simulink model "pmsm"  (R2014b)
settings: Solver=ode45  StartTime=0.0  StopTime=10.0  RelTol=1e-3
undefined symbols (not defined in the file): flux, J, Ld, Lq, Pn, R
settings Model: CovSFcnEnable=on  Creator=Lei  LastModifiedBy=Lei
settings DataIOCC: SignalLoggingSaveFormat=ModelDataLogs  SignalLoggingName=sigsOut
settings DebuggingCC: SaveWithParameterizedLinksMsg=none  UnderspecifiedInitializationDetection=Classic  MergeDetectMultiDrivingBlocksExec=none  SignalResolutionControl=TryResolveAllWithWarning  SolverPrmCheckMsg=none  MultiTaskDSMMsg=warning  MultiTaskCondExecSysMsg=none  FrameProcessingCompatibilityMsg=error  StrictBusMsg=None
settings HardwareCC: TargetUnknown=on
settings GRTTargetCC: CombineOutputUpdateFcns=off  GRTInterface=on

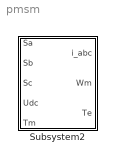
== system pmsm ==
  Subsystem2 : Subsystem

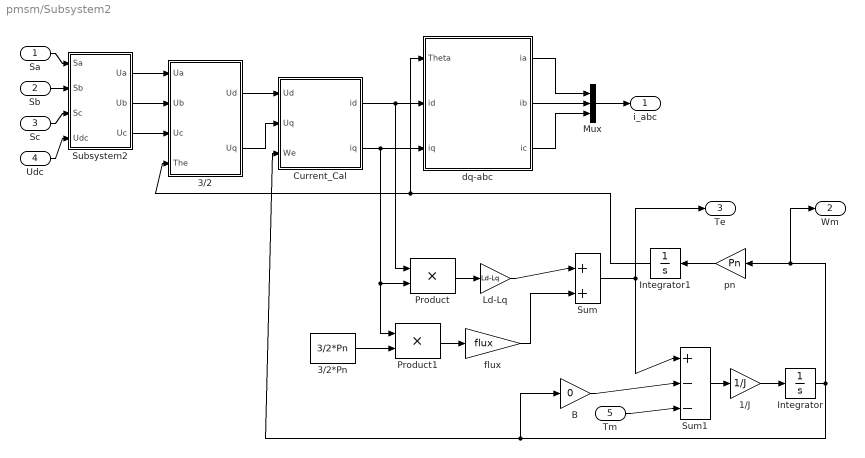
== system pmsm/Subsystem2 ==
  Sa : Inport
  Sb : Inport  Port=2
  Sc : Inport  Port=3
  Udc : Inport  Port=4
  Tm : Inport  Port=5
  1/J : Gain  Gain=1/J  SaturateOnIntegerOverflow=on  OutDataTypeStr=Inherit: Same as input  ParamDataTypeStr=Inherit: Same as input
  3/2 : Subsystem
  3/2*Pn : Constant  Value=3/2*Pn
  B : Gain  Gain=0  SaturateOnIntegerOverflow=on  OutDataTypeStr=Inherit: Same as input  ParamDataTypeStr=Inherit: Same as input
  Current_Cal : Subsystem
  Integrator : Integrator
  Integrator1 : Integrator
  Ld-Lq : Gain  Gain=Ld-Lq  SaturateOnIntegerOverflow=on  OutDataTypeStr=Inherit: Same as input  ParamDataTypeStr=Inherit: Same as input
  Mux : Mux  Inputs=3
  Product : Product  SaturateOnIntegerOverflow=on  OutDataTypeStr=Inherit: Same as first input
  Product1 : Product  SaturateOnIntegerOverflow=on  OutDataTypeStr=Inherit: Same as first input
  Subsystem2 : Subsystem
  Sum : Sum  Inputs=|++  SaturateOnIntegerOverflow=on
  Sum1 : Sum  Inputs=|+--  SaturateOnIntegerOverflow=on
  dq-abc : Subsystem
  flux : Gain  Gain=flux  SaturateOnIntegerOverflow=on  OutDataTypeStr=Inherit: Same as input  ParamDataTypeStr=Inherit: Same as input
  pn : Gain  Gain=Pn  SaturateOnIntegerOverflow=on  OutDataTypeStr=Inherit: Same as input  ParamDataTypeStr=Inherit: Same as input
  i_abc : Outport
  Wm : Outport  Port=2
  Te : Outport  Port=3
  wires:
  Current_Cal/1(id) -> dq-abc/2(id), Product/1
  Current_Cal/2(iq) -> dq-abc/3(iq), Product/2, Product1/1
  3/2/1(Ud) -> Current_Cal/1(Ud)
  3/2/2(Uq) -> Current_Cal/2(Uq)
  Subsystem2/1(Ua) -> 3/2/1(Ua)
  Subsystem2/2(Ub) -> 3/2/2(Ub)
  Subsystem2/3(Uc) -> 3/2/3(Uc)
  Product/1 -> Ld-Lq/1
  Ld-Lq/1 -> Sum/1
  Product1/1 -> flux/1
  3/2*Pn/1 -> Product1/2
  flux/1 -> Sum/2
  Sum/1 -> Sum1/1, Te/1
  Tm/1 -> Sum1/3
  B/1 -> Sum1/2
  Sum1/1 -> 1/J/1
  1/J/1 -> Integrator/1
  Integrator/1 -> Current_Cal/3(We), B/1, pn/1, Wm/1
  Integrator1/1 -> 3/2/4(The), dq-abc/1(Theta)
  pn/1 -> Integrator1/1
  dq-abc/1(ia) -> Mux/1
  dq-abc/2(ib) -> Mux/2
  dq-abc/3(ic) -> Mux/3
  Mux/1 -> i_abc/1
  Sb/1 -> Subsystem2/2(Sb)
  Sc/1 -> Subsystem2/3(Sc)
  Udc/1 -> Subsystem2/4(Udc)
  Sa/1 -> Subsystem2/1(Sa)

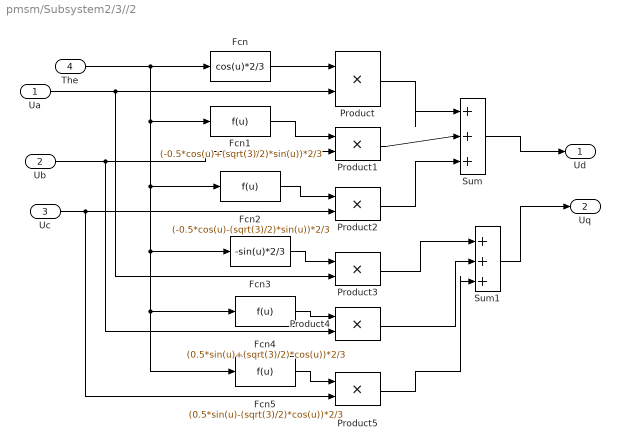
== system pmsm/Subsystem2/3//2 ==
  Ua : Inport
  Ub : Inport  Port=2
  Uc : Inport  Port=3
  The : Inport  Port=4
  Fcn : Fcn  Expr=cos(u)*2/3
  Fcn1 : Fcn  Expr=(-0.5*cos(u)+(sqrt(3)/2)*sin(u))*2/3
  Fcn2 : Fcn  Expr=(-0.5*cos(u)-(sqrt(3)/2)*sin(u))*2/3
  Fcn3 : Fcn  Expr=-sin(u)*2/3
  Fcn4 : Fcn  Expr=(0.5*sin(u)+(sqrt(3)/2)*cos(u))*2/3
  Fcn5 : Fcn  Expr=(0.5*sin(u)-(sqrt(3)/2)*cos(u))*2/3
  Product{,1..5} (6 alike) : Product  SaturateOnIntegerOverflow=on  OutDataTypeStr=Inherit: Same as first input
  Sum : Sum  Inputs=|+++  SaturateOnIntegerOverflow=on
  Sum1 : Sum  Inputs=|+++  SaturateOnIntegerOverflow=on
  Ud : Outport
  Uq : Outport  Port=2
  wires:
  Product/1 -> Sum/1
  Product1/1 -> Sum/2
  Product4/1 -> Sum1/2
  Product5/1 -> Sum1/3
  Sum/1 -> Ud/1
  Fcn/1 -> Product/1
  The/1 -> Fcn1/1, Fcn2/1, Fcn3/1, Fcn5/1, Fcn4/1, Fcn/1
  Ua/1 -> Product/2, Product3/2
  Fcn1/1 -> Product1/1
  Ub/1 -> Product1/2, Product4/2
  Product2/1 -> Sum/3
  Uc/1 -> Product2/2, Product5/2
  Fcn2/1 -> Product2/1
  Sum1/1 -> Uq/1
  Product3/1 -> Sum1/1
  Fcn3/1 -> Product3/1
  Fcn4/1 -> Product4/1
  Fcn5/1 -> Product5/1

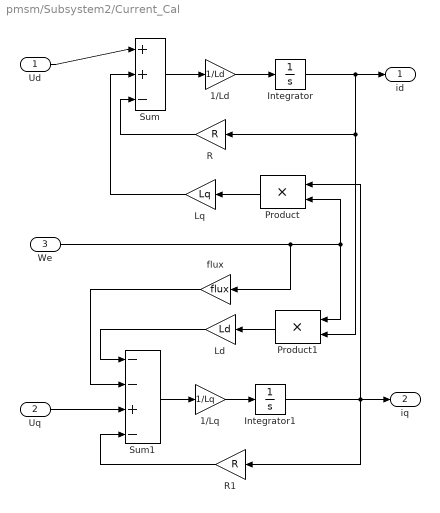
== system pmsm/Subsystem2/Current_Cal ==
  Ud : Inport
  Uq : Inport  Port=2
  We : Inport  Port=3
  1/Ld : Gain  Gain=1/Ld  SaturateOnIntegerOverflow=on  OutDataTypeStr=Inherit: Same as input  ParamDataTypeStr=Inherit: Same as input
  1/Lq : Gain  Gain=1/Lq  SaturateOnIntegerOverflow=on  OutDataTypeStr=Inherit: Same as input  ParamDataTypeStr=Inherit: Same as input
  Integrator : Integrator  InitialCondition=0.01
  Integrator1 : Integrator
  Ld : Gain  Gain=Ld  SaturateOnIntegerOverflow=on  OutDataTypeStr=Inherit: Same as input  ParamDataTypeStr=Inherit: Same as input
  Lq : Gain  Gain=Lq  SaturateOnIntegerOverflow=on  OutDataTypeStr=Inherit: Same as input  ParamDataTypeStr=Inherit: Same as input
  Product : Product  SaturateOnIntegerOverflow=on  OutDataTypeStr=Inherit: Same as first input
  Product1 : Product  SaturateOnIntegerOverflow=on  OutDataTypeStr=Inherit: Same as first input
  R : Gain  Gain=R  SaturateOnIntegerOverflow=on  OutDataTypeStr=Inherit: Same as input  ParamDataTypeStr=Inherit: Same as input
  R1 : Gain  Gain=R  SaturateOnIntegerOverflow=on  OutDataTypeStr=Inherit: Same as input  ParamDataTypeStr=Inherit: Same as input
  Sum : Sum  Inputs=|++-  SaturateOnIntegerOverflow=on
  Sum1 : Sum  Inputs=--+-  SaturateOnIntegerOverflow=on
  flux : Gain  Gain=flux  SaturateOnIntegerOverflow=on  OutDataTypeStr=Inherit: Same as input  ParamDataTypeStr=Inherit: Same as input
  id : Outport
  iq : Outport  Port=2
  wires:
  Ud/1 -> Sum/1
  Sum/1 -> 1/Ld/1
  1/Ld/1 -> Integrator/1
  Integrator/1 -> Product1/2, R/1, id/1
  Product/1 -> Lq/1
  Lq/1 -> Sum/2
  We/1 -> Product/2, Product1/1, flux/1
  R/1 -> Sum/3
  R1/1 -> Sum1/4
  1/Lq/1 -> Integrator1/1
  Sum1/1 -> 1/Lq/1
  Integrator1/1 -> R1/1, Product/1, iq/1
  Product1/1 -> Ld/1
  Ld/1 -> Sum1/1
  Uq/1 -> Sum1/3
  flux/1 -> Sum1/2

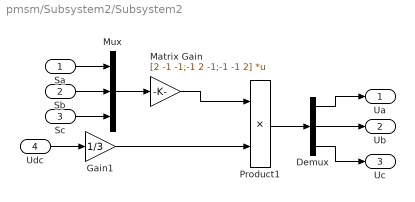
== system pmsm/Subsystem2/Subsystem2 ==
  Sa : Inport
  Sb : Inport  Port=2
  Sc : Inport  Port=3
  Udc : Inport  Port=4
  Demux : Demux  Outputs=3
  Gain1 : Gain  Gain=1/3  SaturateOnIntegerOverflow=on  OutDataTypeStr=Inherit: Same as input  ParamDataTypeStr=Inherit: Same as input
  Matrix Gain : Gain  Gain=[2 -1 -1;-1 2 -1;-1 -1 2]  Multiplication=Matrix(K*u)  SaturateOnIntegerOverflow=on  OutDataTypeStr=Inherit: Same as input  ParamDataTypeStr=Inherit: Same as input
  Mux : Mux  Inputs=3
  Product1 : Product  SaturateOnIntegerOverflow=on  OutDataTypeStr=Inherit: Same as first input
  Ua : Outport
  Ub : Outport  Port=2
  Uc : Outport  Port=3
  wires:
  Mux/1 -> Matrix Gain/1
  Matrix Gain/1 -> Product1/1
  Gain1/1 -> Product1/2
  Product1/1 -> Demux/1
  Demux/1 -> Ua/1
  Demux/2 -> Ub/1
  Demux/3 -> Uc/1
  Sa/1 -> Mux/1
  Sb/1 -> Mux/2
  Sc/1 -> Mux/3
  Udc/1 -> Gain1/1

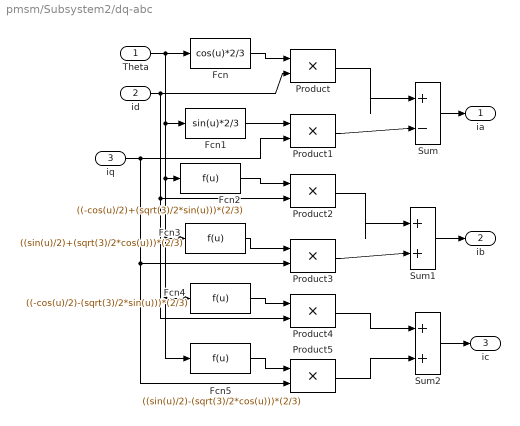
== system pmsm/Subsystem2/dq-abc ==
  Theta : Inport
  id : Inport  Port=2
  iq : Inport  Port=3
  Fcn : Fcn  Expr=cos(u)*2/3
  Fcn1 : Fcn  Expr=sin(u)*2/3
  Fcn2 : Fcn  Expr=((-cos(u)/2)+(sqrt(3)/2*sin(u)))*(2/3)
  Fcn3 : Fcn  Expr=((sin(u)/2)+(sqrt(3)/2*cos(u)))*(2/3)
  Fcn4 : Fcn  Expr=((-cos(u)/2)-(sqrt(3)/2*sin(u)))*(2/3)
  Fcn5 : Fcn  Expr=((sin(u)/2)-(sqrt(3)/2*cos(u)))*(2/3)
  Product{,1..5} (6 alike) : Product  SaturateOnIntegerOverflow=on  OutDataTypeStr=Inherit: Same as first input
  Sum : Sum  Inputs=|+-  SaturateOnIntegerOverflow=on
  Sum1 : Sum  Inputs=|++  SaturateOnIntegerOverflow=on
  Sum2 : Sum  SaturateOnIntegerOverflow=on
  ia : Outport
  ib : Outport  Port=2
  ic : Outport  Port=3
  wires:
  Fcn/1 -> Product/1
  Theta/1 -> Fcn5/1, Fcn4/1, Fcn3/1, Fcn2/1, Fcn1/1, Fcn/1
  id/1 -> Product4/2, Product2/2, Product/2
  Product/1 -> Sum/1
  Fcn1/1 -> Product1/1
  Product1/1 -> Sum/2
  iq/1 -> Product3/2, Product5/2, Product1/2
  Sum/1 -> ia/1
  Fcn2/1 -> Product2/1
  Fcn3/1 -> Product3/1
  Fcn5/1 -> Product5/1
  Fcn4/1 -> Product4/1
  Product2/1 -> Sum1/1
  Product3/1 -> Sum1/2
  Product4/1 -> Sum2/1
  Product5/1 -> Sum2/2
  Sum2/1 -> ic/1
  Sum1/1 -> ib/1
